simulink model "bustest"  (R2018a)
settings: Solver=VariableStepAuto  StartTime=0.0  StopTime=10.0  RelTol=1e-3
undefined symbols (not defined in the file or in its folder): BaseVoltage, ControlModes, ILDC, m, n, RCReg1, Reg1i, Reg1v, TReg1
(part 2 of 2)

== stateflow chart bustest/Action Coordinator ==
  state Asleep
  state SendingRegCtrlAction
    en:OutputAction.data = ...
    RegCtrlAction.data;
    send(OutputAction);
  state SendingSolverAction
    en:OutputAction.data = ...
    SolverAction.data;
    send(SolverAction);
  state SendingExecAction
    en:OutputAction.data = ...
    ExecAction.data;
    send(OutputAction);
  (default) -> Asleep
  Asleep -> SendingRegCtrlAction [order 1] : RegCtrlAction
  Asleep -> SendingSolverAction [order 3] : SolverAction
  SendingSolverAction -> Asleep
  SendingRegCtrlAction -> Asleep
  Asleep -> SendingExecAction [order 2] : ExecAction
  SendingExecAction -> Asleep
  data: RegCtrlAction input Enum: QueueActions; ExecAction input Enum: QueueActions; SolverAction input Enum: QueueActions; OutputAction output Enum: QueueActions

== stateflow chart bustest/Queue Handler ==
  settings: enableNonTerminalStates=1
  state Executive [parallel]
    settings: executionOrder=1
    state Asleep
      ex: Status.data = Statuses.READY; % reset status
      INTERNAL_DONE = false;
      EXECUTIVE_DONE = false;
    state DoNearestActions
      state WaitOnPeek
        en: send(QUEUE_PEEK, Internal);
      state WaitOnPop
        en: send(QUEUE_POP, Internal);
      state ErrorNoItems
        en: Status.data = ...
        Statuses.ERROR;
        send(Status);
      (default) -> (junction 302) : % do only those actions with the same delay time as the first action time return time
          | {q_len_initial = GetQueueSize;
          | PendingActionsCompleted = false; % local for now
          | }
      (junction 302) -> (junction 315) [order 1] : [q_len_initial > 0]
      (junction 302) -> Executive.DoNearestActions.ErrorNoItems [order 2]
      (junction 315) -> WaitOnPeek : {INTERNAL_DONE = false;
          | ActionTime = ExternalAT; % peek with given AT
          | }
      (junction 301) -> (junction 331) [order 1] : [jj <= q_len_initial]
      (junction 331) -> Executive.DoNearestActions.WaitOnPop : {INTERNAL_DONE = false;}
      WaitOnPeek -> (junction 301) : [INTERNAL_DONE]
          | {ActionTime = Out(QF.Time);
          | QHour = Out(QF.Hour);
          | QSec = Out(QF.Sec);
          | jj = 1;}
      Executive.DoNearestActions.WaitOnPop -> (junction 299) : [INTERNAL_DONE]
          | %send(DoPendingAction);
      (junction 299) -> (junction 301) : {jj = jj + 1;}
      (junction 301) -> (junction 305) [order 2]
      Executive.DoNearestActions.ErrorNoItems -> (junction 300)
      (junction 305) -> (junction 300)
      (junction 300) -> (junction 298) : {EXECUTIVE_DONE = true;}
    state DoAllActions
      state WaitOnPop
        en: send(QUEUE_POP, Internal);
      state ErrorNoItems
        en: Status.data = ...
        Statuses.ERROR;
        send(Status);
      (default) -> (junction 322) : {q_len_initial = GetQueueSize;}
      (junction 322) -> (junction 321) [order 1] : [q_len_initial ~= 0]
      (junction 322) -> Executive.DoAllActions.ErrorNoItems [order 2]
      (junction 321) -> (junction 326) : {ActionTime = ExternalAT;
          | jj = 1;}
      (junction 326) -> (junction 316) [order 1] : [jj <= q_len_initial]
      (junction 316) -> Executive.DoAllActions.WaitOnPop : {INTERNAL_DONE = false;}
      (junction 314) -> (junction 326) : {jj = jj + 1;}
      (junction 326) -> (junction 312) [order 2]
      Executive.DoAllActions.WaitOnPop -> (junction 314) : [INTERNAL_DONE]
          | %send(DoPendingAction);
      Executive.DoAllActions.ErrorNoItems -> (junction 324)
      (junction 312) -> (junction 324)
      (junction 324) -> (junction 310) : {EXECUTIVE_DONE = true;}
    state Pushing
      en: send(QUEUE_PUSH, Internal);
    state DeletingByHandle
      en: send(QUEUE_DELETE, Internal);
    state Peeking
      en: send(QUEUE_PEEK, Internal);
    state Popping
      en: send(QUEUE_POP, Internal);
    state ReadyAgain
      Status.data = Statuses.READY;
      send(Status);
    Executive.Asleep -> Executive.DeletingByHandle [order 6] : QueueAction[QueueAction.data == ...
        | QueueActions.DELETE]
    Executive.Asleep -> Executive.Peeking [order 5] : QueueAction[QueueAction.data == ...
        | QueueActions.PEEK]
    Executive.Asleep -> Executive.Popping [order 4] : QueueAction[QueueAction.data == ...
        | QueueActions.POP]
    (default) -> Executive.Asleep
    Executive.Asleep -> Executive.Pushing [order 3] : QueueAction[QueueAction.data == ...
        | QueueActions.PUSH]
    Executive.Asleep -> DoAllActions [order 2] : QueueAction[QueueAction.data == ...
        | QueueActions.DO_ALL_ACTIONS]
    ReadyAgain -> Executive.Asleep
    Executive.Asleep -> DoNearestActions [order 1] : QueueAction[QueueAction.data == DO_NEAREST_ACTIONS]
    Executive.Pushing -> ReadyAgain : [INTERNAL_DONE]
    Executive.Popping -> ReadyAgain : [INTERNAL_DONE]
    Executive.DeletingByHandle -> ReadyAgain : [INTERNAL_DONE]
    Executive.Peeking -> ReadyAgain : [INTERNAL_DONE]
    DoAllActions -> ReadyAgain : [EXECUTIVE_DONE]
    DoNearestActions -> ReadyAgain : [EXECUTIVE_DONE]
  state Internal [parallel]
    settings: executionOrder=2
    state Asleep
    state Popping
      (default) -> (junction 163) : % delete from beginning, t<= ActionTime:
          | {q_len = GetQueueSize;
          | ii = 1;
          | }
      (junction 163) -> (junction 169) [order 1] : [ii <= q_len]
      (junction 169) -> (junction 157)
      (junction 157) -> (junction 158) [order 1] : [GetElemTime(ii) <= ActionTime]
      (junction 157) -> (junction 164) [order 2]
      (junction 158) -> (junction 159) : {Out = GetElem(ii);
          | ReduceQueue(ii);
          | send(DoPendingAction);}
          | % break
      (junction 164) -> (junction 163) : {ii = ii + 1;}
      (junction 163) -> (junction 165) [order 2]
      (junction 159) -> (junction 165)
      (junction 165) -> (junction 640)
      (junction 640) -> (junction 641) [order 1] : [QueueEmpty.data == true]
      (junction 640) -> (junction 642) [order 2]
      (junction 641) -> (junction 643) : {send(QueueEmpty);}
      (junction 643) -> (junction 642)
      (junction 642) -> (junction 644) : {INTERNAL_DONE = true;}
    state DeletingByHandle
      (default) -> (junction 664) : % delete from beginning, t<= ActionTime:
          | {q_len = GetQueueSize;
          | ii = 1;
          | }
      (junction 664) -> (junction 671) [order 1] : [ii <= q_len]
      (junction 671) -> (junction 670)
      (junction 670) -> (junction 665) [order 1] : [GetElemHandle(ii) == ExternalHandle]
      (junction 670) -> (junction 663) [order 2]
      (junction 665) -> (junction 660) : {Out = GetElem(ii);
          | ReduceQueue(ii);}
          | % break
      (junction 663) -> (junction 664) : {ii = ii + 1;}
      (junction 664) -> (junction 668) [order 2]
      (junction 660) -> (junction 668)
      (junction 668) -> (junction 666)
      (junction 666) -> (junction 658) [order 1] : [QueueEmpty.data == true]
      (junction 666) -> (junction 661) [order 2]
      (junction 658) -> (junction 667) : {send(QueueEmpty);}
      (junction 667) -> (junction 661)
      (junction 661) -> (junction 655) : {INTERNAL_DONE = true;}
    state Pushing
      (default) -> (junction 136) : % insert into queue right before item of greater or equal execution time
          | {q_cand = In'; % transposition to 1 x 5
          | q_len = GetQueueSize; %size(queue, 3);
          | ii = 1;
          | }
      (junction 136) -> (junction 134) [order 1] : [ii <= q_len]
      (junction 134) -> (junction 145)
      (junction 145) -> (junction 146) [order 1] : [q_cand(1,QF.Time) <= GetElemTime(ii)]
      (junction 145) -> (junction 137) [order 2]
      (junction 146) -> (junction 148) : {
          | ExpandQueue(ii);}
          | % break
      (junction 137) -> (junction 136) : {ii = ii + 1;}
      (junction 136) -> (junction 138) [order 2] : {ExpandQueue(q_len+1);}
      (junction 148) -> (junction 138)
      (junction 138) -> (junction 151) : %{send(DONE_PUSHING, Executive.Pushing);}
          | {INTERNAL_DONE = true;}
    state Peeking
      (default) -> (junction 181) : % pop without deletion
          | {q_len = GetQueueSize;
          | ii = 1;
          | }
      (junction 181) -> (junction 187) [order 1] : [ii <= q_len]
      (junction 187) -> (junction 175)
      (junction 175) -> (junction 176) [order 1] : [GetElemTime(ii) <= ActionTime]
      (junction 175) -> (junction 182) [order 2]
      (junction 176) -> (junction 177) : {Out = GetElem(ii);}
          | % break
      (junction 182) -> (junction 181) : {ii = ii + 1;}
      (junction 181) -> (junction 183) [order 2]
      (junction 177) -> (junction 183)
      (junction 183) -> (junction 180) : {INTERNAL_DONE = true;}
    (default) -> Internal.Asleep
    Internal.Asleep -> Internal.Pushing [order 1] : QUEUE_PUSH
    Internal.Pushing -> Internal.Asleep : [INTERNAL_DONE]
    Internal.Asleep -> Internal.Popping [order 2] : QUEUE_POP
    Internal.Popping -> Internal.Asleep : [INTERNAL_DONE]
    Internal.Asleep -> Internal.Peeking [order 3] : QUEUE_PEEK
    Internal.Peeking -> Internal.Asleep : [INTERNAL_DONE]
    Internal.Asleep -> Internal.DeletingByHandle [order 4] : QUEUE_DELETE
    Internal.DeletingByHandle -> Internal.Asleep : [INTERNAL_DONE]
  state QF % Queue Fields [group]
  data: Handle local double =1; Time local double =2; Hour local double =3; Sec local double =4; ActionCode local double =5; depth function_input; h function_output; qs function_output; depth function_input; et function_output; elem function_output; depth function_input; depth function_input; depth function_input; DoPendingAction output boolean =true; QueueAction input Enum: QueueActions; Status output Enum: Statuses; Out output double size=[1 5]; queue output double size=[1 5 50]; q_len local double =0; PendingActionsCompleted local boolean =false; QHour local double; QSec local double; q_cand local double size=[1 5]; In input double size=5; qwriteflag local boolean =false; ii local uint8; jj local uint8; q_len_initial local double; EXECUTIVE_DONE local boolean =false; INTERNAL_DONE local boolean =false;; ExternalAT input double =100; ActionTime local double; QueueEmpty output boolean =false; ExternalHandle input uint8
  events: QUEUE_POP local FUNCTION_CALL_EVENT; QUEUE_PUSH local FUNCTION_CALL_EVENT; QUEUE_PEEK local FUNCTION_CALL_EVENT; QUEUE_DELETE local FUNCTION_CALL_EVENT
  function h = GetElemHandle(depth):
    | function h = GetElemHandle(depth)
    |     h = zeros(1,1);
    |     if ~isempty(queue)
    |         h = queue(1,QF.Handle,ii);
    |         h = cast(h, 'uint8'); % for comparison with ExternalHandle
    |     else
    | end
  function qs = GetQueueSize:
    | function qs = GetQueueSize
    | %     coder.extrinsic('exist');
    | %     eq = zeros(1,1,'double');
    | %     eq = exist('queue');
    | %     if eq == 1 && ~isempty(queue)
    | %         qs = size(queue, 3);
    | %     else % eq ~= 1 || size == 0
    | %         qs = 0;
    | %     end
    |     if ~qwriteflag % can't read intial value of empty queue, so depend on flag
    |         queue = zeros(1,5);
    |         qs = 0;
    |         QueueEmpty.data = true;
    |         qwriteflag = true;
    |     elseif isequal(queue,zeros(1,5)) % case of empty queue (still 1 element)
    |         qs = 0;
    |         QueueEmpty.data = true;
    |     else
    |         qs = size(queue,3);
    |         QueueEmpty.data = false;
    |     end
    | end
  function et = GetElemTime(depth):
    | function et = GetElemTime(depth)
    |     et = zeros(1,1);
    |     if ~isempty(queue)
    |         et = queue(1,QF.Time,ii);
    |     else
    |     end
    | end
  function elem = GetElem(depth):
    | function elem = GetElem(depth)
    |     elem = zeros(1,5);
    |     elem(1,:) = queue(:,:,depth);
    | end
  function ExpandQueue(depth):
    | function ExpandQueue(depth)
    |     rhs = queue(:,:,depth:q_len); % the RHS of the queue
    |     bigger = zeros(1,5,q_len+1);
    |     bigger(:,:,1:(depth-1)) = queue(:,:,1:(depth-1)); % copy LHS
    |     bigger(:,:,depth) = q_cand; % inserting element at end of LHS
    |     %queue(:,:,depth) = q_cand; 
    |     bigger(:,:, (depth+1):(q_len+1)) = rhs; % tack on RHS again
    |     queue = bigger;
    | end
  function ReduceQueue(depth):
    | function ReduceQueue(depth)
    |     rhs = queue(:,:,(depth+1):q_len); % excluding element at depth
    |     smaller = zeros(1,5,q_len-1);
    |     smaller(:,:,1:(depth-1)) = queue(:,:,1:(depth-1)); % lhs, excl. depth
    |     smaller(:,:,depth:(q_len-1)) = rhs; % tack on rhs
    |     queue = smaller;
    | end
